simulink model "Q7_Simulink"  (R2019a)
settings: Solver=VariableStepAuto  StartTime=0.0  StopTime=simTime  RelTol=1e-3
undefined symbols (not defined in the file or in its folder): f_m, f_m_time, G_y1_d, G_y2_d, G_y3_d, sigma_1, switch_fault, T_s
settings Model: Creator=mfust  LastModifiedBy=Ian

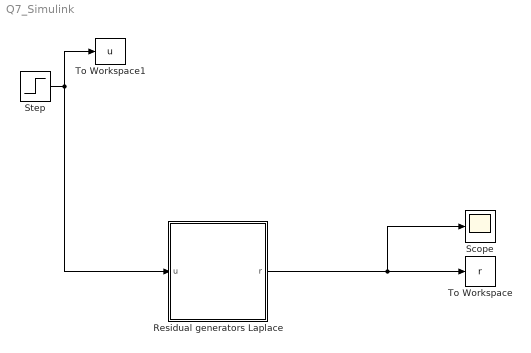
== system Q7_Simulink ==
  Residual generators Laplace : Subsystem
  Scope : Scope
  Step : Step  Time=2  SampleTime=0
  "To Workspace " : ToWorkspace  VariableName=r  SaveFormat=Structure With Time  SampleTime=-1
  To Workspace1 : ToWorkspace  VariableName=u  SaveFormat=Structure With Time  SampleTime=-1
  wires:
  Step/1 -> Residual generators Laplace/1(u), To Workspace1/1
  Residual generators Laplace/1(r) -> Scope/1, "To Workspace "/1

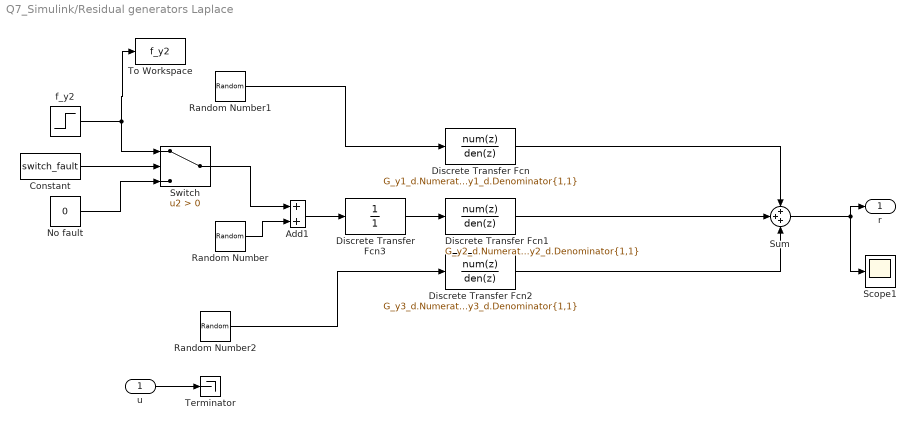
== system Q7_Simulink/Residual generators Laplace ==
  u : Inport
  Add1 : Sum
  Constant : Constant  Value=switch_fault
  Discrete Transfer Fcn : DiscreteTransferFcn  Numerator=G_y1_d.Numerator{1,1}  Denominator=G_y1_d.Denominator{1,1}
  Discrete Transfer Fcn1 : DiscreteTransferFcn  Numerator=G_y2_d.Numerator{1,1}  Denominator=G_y2_d.Denominator{1,1}
  Discrete Transfer Fcn2 : DiscreteTransferFcn  Numerator=G_y3_d.Numerator{1,1}  Denominator=G_y3_d.Denominator{1,1}
  Discrete Transfer Fcn3 : DiscreteTransferFcn  Denominator=[1]  SampleTime=0.004
  No fault : Constant  Value=0
  Random Number : RandomNumber  Variance=sigma_1^2  Seed=325  SampleTime=T_s
  Random Number1 : RandomNumber  Variance=sigma_1^2  Seed=2354363  SampleTime=T_s
  Random Number2 : RandomNumber  Variance=sigma_1^2  Seed=124  SampleTime=T_s
  Scope1 : Scope
  Sum : Sum  Inputs=+++
  Switch : Switch  Criteria=u2 > Threshold
  Terminator : Terminator
  To Workspace : ToWorkspace  VariableName=f_y2  SaveFormat=Structure With Time  SampleTime=-1
  "f_y2 " : Step  Time=f_m_time  After=f_m  SampleTime=0
  r : Outport
  wires:
  Sum/1 -> r/1, Scope1/1
  u/1 -> Terminator/1
  Random Number1/1 -> Discrete Transfer Fcn/1
  Random Number2/1 -> Discrete Transfer Fcn2/1
  Discrete Transfer Fcn1/1 -> Sum/2
  Discrete Transfer Fcn/1 -> Sum/1
  Discrete Transfer Fcn2/1 -> Sum/3
  Random Number/1 -> Add1/2
  Add1/1 -> Discrete Transfer Fcn3/1
  Discrete Transfer Fcn3/1 -> Discrete Transfer Fcn1/1
  "f_y2 "/1 -> Switch/1, To Workspace/1
  No fault/1 -> Switch/3
  Constant/1 -> Switch/2
  Switch/1 -> Add1/1
